simulink model "exemplo_bloco_controle_PID"  (R2024b)
settings: Solver=ode45  StartTime=0.0  StopTime=200.0  RelTol=1e-3  EnableMultiTasking=on
undefined symbols (not defined in the file): MODEL
settings Model: Creator=Mauricio  LastModifiedBy=johne
settings SolverCC: AlgebraicLoopSolver=TrustRegion
settings DataIOCC: LimitDataPoints=on  SaveFormat=Array  ReturnWorkspaceOutputs=off
settings OptimizationCC: InitFltsAndDblsToZero=on  LifeSpan=inf
settings DebuggingCC: SaveWithParameterizedLinksMsg=none  SignalResolutionControl=TryResolveAllWithWarning  SolverPrmCheckMsg=warning  MultiTaskDSMMsg=warning  MultiTaskCondExecSysMsg=none  FcnCallInpInsideContextMsg=warning  UnconnectedInputMsg=warning  UnconnectedOutputMsg=warning  UnconnectedLineMsg=warning  SFUnexpectedBacktrackingDiag=warning  SFNoUnconditionalDefaultTransitionDiag=warning  SFExecutionAtInitializationDiag=none  ArithmeticOperatorsInVariantConditions=warning
settings HardwareCC: ProdBitPerPointer=32  ProdBitPerSizeT=32  ProdBitPerPtrDiffT=32  ProdLargestAtomicFloat=None  ProdIntDivRoundTo=Undefined  ProdEndianess=Unspecified  ProdWordSize=32  ProdHWDeviceType=32-bit Generic
settings ModelReferenceCC: EnableRefExpFcnMdlSchedulingChecks=on  PropagateSignalLabelsOutOfModel=off
settings SFSimCC: SimUseLocalCustomCode=off  CustomCodeUndefinedFunction=UseInterfaceOnly
settings RTWCC: RTWUseLocalCustomCode=off  GPUComputeCapability=3.5
settings CodeAppCC: StateflowObjectComments=on
settings GRTTargetCC: TargetFcnLib=ansi_tfl_tmw.mat  TargetLangStandard=C89/C90 (ANSI)  CombineOutputUpdateFcns=off  GRTInterface=on
settings ConfigComp: CovMetricSettings=dw  CovSaveCumulativeToWorkspaceVar=on  CovSaveSingleToWorkspaceVar=on  CovExternalEMLEnable=off  CovSFcnEnable=off

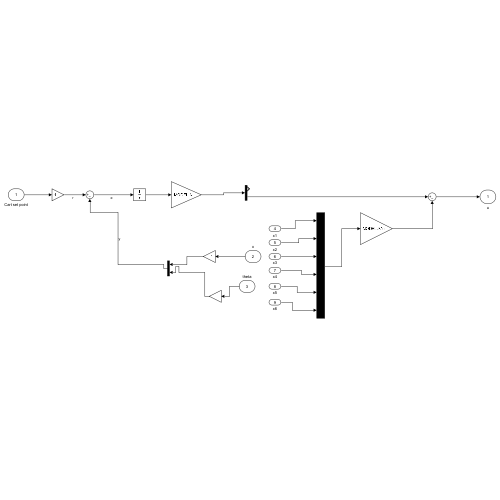
[thumbnail: Simulink's stored preview of the top-level diagram]
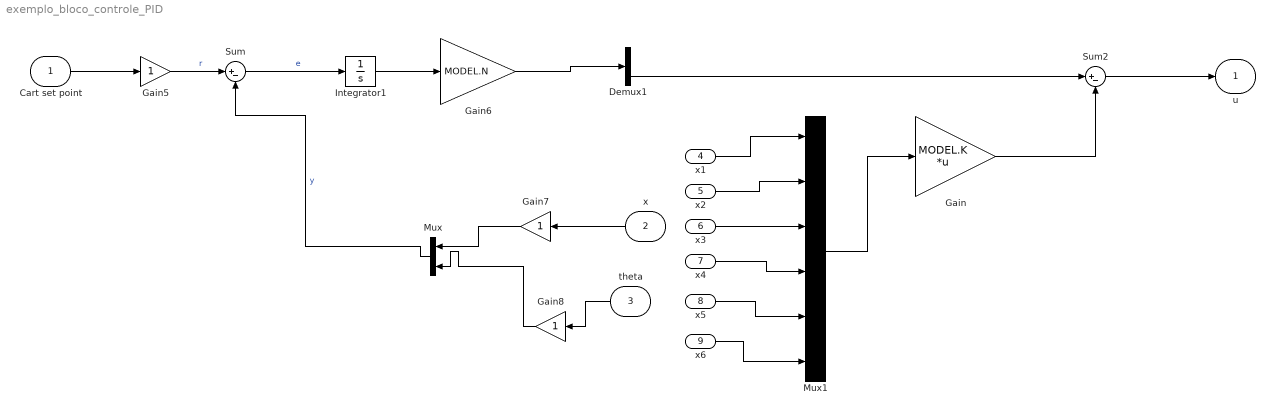
== system exemplo_bloco_controle_PID ==
  Cart set point : Inport
  x : Inport  Port=2
  theta : Inport  Port=3
  x1 : Inport  Port=4
  x2 : Inport  Port=5
  x3 : Inport  Port=6
  x4 : Inport  Port=7
  x5 : Inport  Port=8
  x6 : Inport  Port=9
  Demux1 : Demux  Outputs=2
  Gain : Gain  Gain=MODEL.K  Multiplication=Matrix(K*u)
  Gain5 : Gain
  Gain6 : Gain  Gain=MODEL.N
  Gain7 : Gain
  Gain8 : Gain
  Integrator1 : Integrator
  Mux : Mux  Inputs=2
  Mux1 : Mux  Inputs=6
  Sum : Sum  Inputs=|+-
  Sum2 : Sum  Inputs=|+-
  u : Outport  VectorParamsAs1DForOutWhenUnconnected=off
  wires:
  Gain7/1 -> Mux/1
  Gain5/1 -> Sum/1  "r"
  theta/1 -> Gain8/1
  x4/1 -> Mux1/4
  Mux/1 -> Sum/2  "y"
  x3/1 -> Mux1/3
  x1/1 -> Mux1/1
  x2/1 -> Mux1/2
  Gain8/1 -> Mux/2
  x6/1 -> Mux1/6
  x5/1 -> Mux1/5
  Gain6/1 -> Demux1/1
  Sum/1 -> Integrator1/1  "e"
  x/1 -> Gain7/1
  Cart set point/1 -> Gain5/1
  Integrator1/1 -> Gain6/1
  Gain/1 -> Sum2/2
  Demux1/2 -> Sum2/1
  Sum2/1 -> u/1
  Mux1/1 -> Gain/1
